simulink model "SSB"  (R2020b)
settings: Solver=VariableStepAuto  StartTime=0.0  StopTime=0.005  RelTol=1e-3
libraries: dsparch4 x3
settings Model: Creator=LENOVO  LastModifiedBy=LENOVO

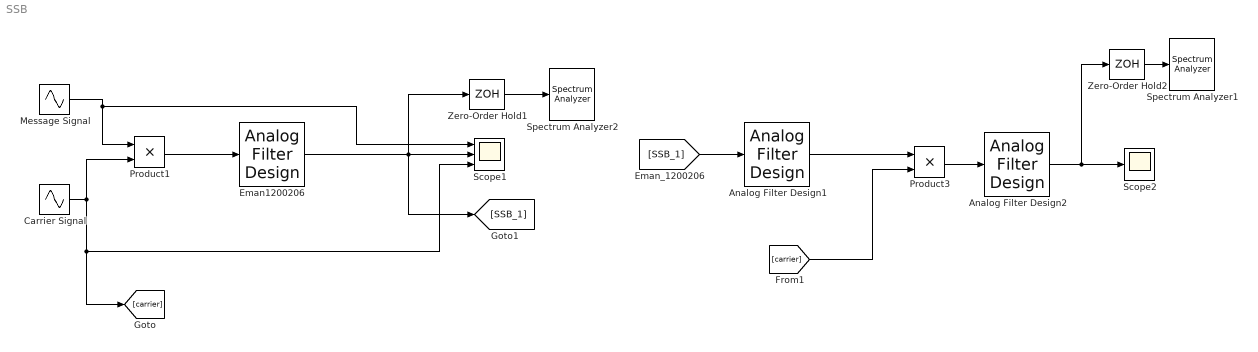
== system SSB ==
  Analog Filter Design1 : dsparch4/Analog Filter Design  method=Butterworth  filttype=Bandpass  N=2  Wlo=13000*2*pi  Whi=15000*2*pi  Rp=2  Rs=40
  Analog Filter Design2 : dsparch4/Analog Filter Design  method=Butterworth  filttype=Lowpass  N=2  Wlo=1000*2*pi  Whi=3000*2*pi  Rp=2  Rs=40
  Carrier Signal : Sin  Frequency=15000*pi*2  Phase=90*pi*2  SampleTime=0
  Eman1200206 : dsparch4/Analog Filter Design  method=Butterworth  filttype=Bandpass  N=2  Wlo=15000*2*pi  Whi=17000*2*pi  Rp=2  Rs=40
  Message Signal : Sin  Amplitude=0.85  Frequency=1000*pi*2  Phase=90*pi*2  SampleTime=0
  Product1 : Product
  Product3 : Product
  Scope1 : Scope  NumInputPorts=3
  Scope2 : Scope
  Spectrum Analyzer1 : SpectrumAnalyzer
  Spectrum Analyzer2 : SpectrumAnalyzer
  Zero-Order Hold1 : ZeroOrderHold  SampleTime=-1
  Zero-Order Hold2 : ZeroOrderHold  SampleTime=-1
  wires:
  Message Signal/1 -> Scope1/1, Product1/1
  Carrier Signal/1 -> Product1/2, [carrier], Scope1/3
  Product1/1 -> Eman1200206/1
  [SSB_1] -> Analog Filter Design1/1
  [carrier] -> Product3/2
  Analog Filter Design1/1 -> Product3/1
  Product3/1 -> Analog Filter Design2/1
  Analog Filter Design2/1 -> Zero-Order Hold2/1, Scope2/1
  Zero-Order Hold2/1 -> Spectrum Analyzer1/1
  Zero-Order Hold1/1 -> Spectrum Analyzer2/1
  Eman1200206/1 -> Scope1/2, Zero-Order Hold1/1, [SSB_1]
